simulink model "PD_satellite"  (R2018b)
settings: Solver=VariableStepAuto  StartTime=0.0  StopTime=3  RelTol=1e-3
settings Model: Creator=carlos  LastModifiedBy=carlos

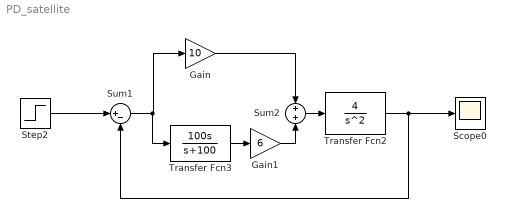
== system PD_satellite ==
  Gain : Gain  Gain=10
  Gain1 : Gain  Gain=6
  Scope0 : Scope
  Step2 : Step  Time=0  SampleTime=0
  Sum1 : Sum  Inputs=|+-
  Sum2 : Sum
  Transfer Fcn2 : TransferFcn  Numerator=4  Denominator=[1 0 0]
  Transfer Fcn3 : TransferFcn  Numerator=[100 0]  Denominator=[1 100]
  wires:
  Step2/1 -> Sum1/1
  Transfer Fcn2/1 -> Sum1/2, Scope0/1
  Sum1/1 -> Transfer Fcn3/1, Gain/1
  Transfer Fcn3/1 -> Gain1/1
  Sum2/1 -> Transfer Fcn2/1
  Gain1/1 -> Sum2/2
  Gain/1 -> Sum2/1
